simulink model "tmp"  (R2020b)
settings: Solver=ode45  StartTime=0.0  StopTime=3  RelTol=1e-4
undefined symbols (not defined in the file): DiscIntNeverNeededParam, sens
libraries: simulink x1
settings Model: Creator=Utente  LastModifiedBy=Utente
settings SolverCC: ZeroCrossAlgorithm=Adaptive
settings DataIOCC: ReturnWorkspaceOutputs=off
settings DebuggingCC: IgnoredZcDiagnostic=none

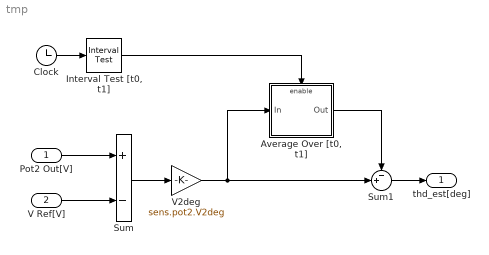
== system tmp ==
  Pot2 Out[V] : Inport
  V Ref[V] : Inport  Port=2
  "Average Over [t0, t1]" : Subsystem
  Clock : Clock
  "Interval Test [t0, t1]" : simulink/Logic and Bit Operations/Interval Test  IntervalClosedRight=on  uplimit=0.7  IntervalClosedLeft=on  lowlimit=0.2  OutDataTypeStr=boolean
  Sum : Sum  Inputs=+-
  Sum1 : Sum  Inputs=-+|
  V2deg : Gain  Gain=sens.pot2.V2deg
  thd_est[deg] : Outport
  wires:
  V Ref[V]/1 -> Sum/2
  Pot2 Out[V]/1 -> Sum/1
  Sum/1 -> V2deg/1
  V2deg/1 -> "Average Over [t0, t1]"/1(In), Sum1/2
  "Average Over [t0, t1]"/1(Out) -> Sum1/1
  Clock/1 -> "Interval Test [t0, t1]"/1
  "Interval Test [t0, t1]"/1 -> "Average Over [t0, t1]"/Enable
  Sum1/1 -> thd_est[deg]/1

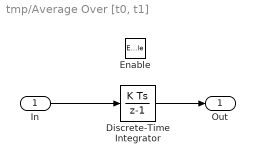
== system tmp/Average Over [t0, t1] ==
  In : Inport
  Enable : EnablePort
  Discrete-Time Integrator : DiscreteIntegrator  SampleTime=-1  ICPrevOutput=DiscIntNeverNeededParam  ICPrevScaledInput=DiscIntNeverNeededParam
  Out : Outport
  wires:
  Discrete-Time Integrator/1 -> Out/1
  In/1 -> Discrete-Time Integrator/1
